simulink model "pts_torque_2"  (Simulink 8.9)
settings: Solver=ode5  StartTime=0.0  StopTime=3.5604  FixedStep=0.005  RelTol=1e-3  AbsTol=1e-6  EnableMultiTasking=on
values from neighbouring files (symbols this model uses):
  Kp = omega.^2    [init_3pts.m]
  kt = [20 7]    [init_3pts.m]
  Kv = 2*chi*omega    [init_3pts.m]
  ListePoints = [130*pi/360 130*pi/360;50*pi/360 90*pi/360; 6*pi/360 60*pi/360]    [init_3pts.m]
undefined symbols (not defined in the file or in its folder): inter_arti_d6, scarabase_ddm, scarabase_dyn
settings Model: SuppressorTable=22 serialization::archive 11 0 6 0 0 0 11 0  Creator=user  LastModifiedBy=steff  ExtModeTrigMode=oneshot  ExtModeArmWhenConnect=off
settings DataIOCC: LimitDataPoints=off  SignalLoggingName=sigsOut
settings OptimizationCC: BooleanDataType=off  ExpressionDepthLimit=2147483647
settings DebuggingCC: SaveWithParameterizedLinksMsg=none  SignalResolutionControl=TryResolveAllWithWarning  MultiTaskDSMMsg=warning  MultiTaskCondExecSysMsg=none
settings HardwareCC: TargetUnknown=on
settings RTWCC: TemplateMakefile=grt_vc.tmf

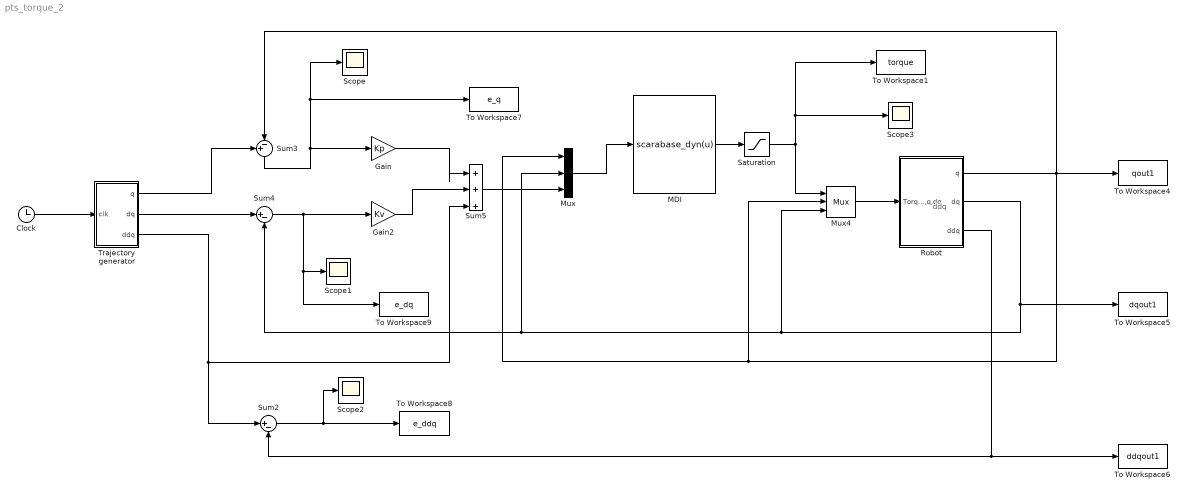
== system pts_torque_2 ==
  note: ddq
  Clock : Clock
  Gain : Gain  Gain=Kp
  Gain2 : Gain  Gain=Kv
  MDI : MATLABFcn  MATLABFcn=scarabase_dyn(u)  OutputDimensions=2  Output1D=off
  Mux : Mux  Inputs=3
  Mux4 : Mux  Inputs=3
  Robot : Subsystem
  Saturation : Saturate  UpperLimit=kt  LowerLimit=-kt
  Scope{,1..3} (4 alike) : Scope
  Sum2 : Sum  Inputs=|+-  SaturateOnIntegerOverflow=on
  Sum3 : Sum  Inputs=+-|  SaturateOnIntegerOverflow=on
  Sum4 : Sum  Inputs=|+-  SaturateOnIntegerOverflow=on
  Sum5 : Sum  Inputs=|+++
  To Workspace1 : ToWorkspace  VariableName=torque  SampleTime=-1
  To Workspace4 : ToWorkspace  VariableName=qout1  SampleTime=-1
  To Workspace5 : ToWorkspace  VariableName=dqout1  SampleTime=-1
  To Workspace6 : ToWorkspace  VariableName=ddqout1  SampleTime=-1
  To Workspace7 : ToWorkspace  VariableName=e_q  SampleTime=-1
  To Workspace8 : ToWorkspace  VariableName=e_ddq  SampleTime=-1
  To Workspace9 : ToWorkspace  VariableName=e_dq  SampleTime=-1
  Trajectory generator : Subsystem
  wires:
  Sum2/1 -> To Workspace8/1, Scope2/1
  Sum3/1 -> Scope/1, To Workspace7/1, Gain/1
  Sum4/1 -> Gain2/1, Scope1/1, To Workspace9/1
  Gain/1 -> Sum5/1
  Gain2/1 -> Sum5/2
  MDI/1 -> Saturation/1
  Mux/1 -> MDI/1
  Saturation/1 -> Mux4/1, To Workspace1/1, Scope3/1
  Sum5/1 -> Mux/3
  Trajectory generator/1(q) -> Sum3/1
  Trajectory generator/3(ddq) -> Sum5/3, Sum2/1
  Trajectory generator/2(dq) -> Sum4/1
  Clock/1 -> Trajectory generator/1(clk)
  Robot/3(ddq) -> Sum2/2, To Workspace6/1
  Robot/2(dq) -> Mux4/3, Mux/2, Sum4/2, To Workspace5/1
  Mux4/1 -> Robot/1(Torque,q,dq)
  Robot/1(q) -> Mux/1, Mux4/2, To Workspace4/1, Sum3/2

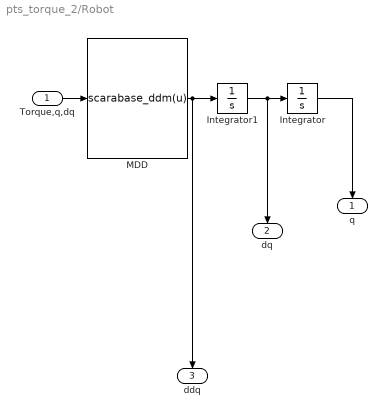
== system pts_torque_2/Robot ==
  Torque,q,dq : Inport
  Integrator : Integrator  InitialCondition=ListePoints(1,:)
  Integrator1 : Integrator  InitialCondition=[0 0]
  MDD : MATLABFcn  MATLABFcn=scarabase_ddm(u)  OutputDimensions=2
  q : Outport
  dq : Outport  Port=2
  ddq : Outport  Port=3
  wires:
  Integrator1/1 -> dq/1, Integrator/1
  Integrator/1 -> q/1
  MDD/1 -> ddq/1, Integrator1/1
  Torque,q,dq/1 -> MDD/1

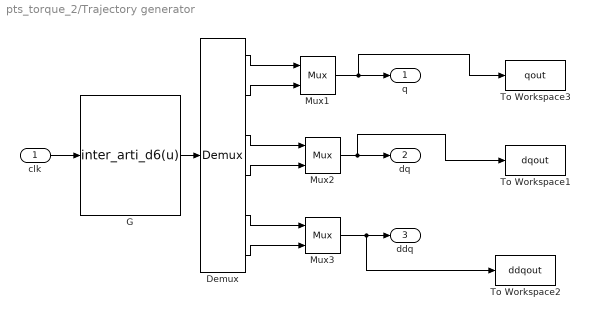
== system pts_torque_2/Trajectory generator ==
  clk : Inport
  Demux : Demux  Outputs=6
  G : MATLABFcn  MATLABFcn=inter_arti_d6(u)  OutputDimensions=6  Output1D=off
  Mux1 : Mux  Inputs=2
  Mux2 : Mux  Inputs=2
  Mux3 : Mux  Inputs=2
  To Workspace1 : ToWorkspace  VariableName=dqout  SampleTime=-1
  To Workspace2 : ToWorkspace  VariableName=ddqout  SampleTime=-1
  To Workspace3 : ToWorkspace  VariableName=qout  SampleTime=-1
  q : Outport
  dq : Outport  Port=2
  ddq : Outport  Port=3
  wires:
  Demux/1 -> Mux1/1
  Demux/6 -> Mux3/2
  Demux/3 -> Mux2/1
  Mux2/1 -> To Workspace1/1, dq/1
  Demux/2 -> Mux1/2
  Demux/4 -> Mux2/2
  Demux/5 -> Mux3/1
  clk/1 -> G/1
  Mux3/1 -> To Workspace2/1, ddq/1
  G/1 -> Demux/1
  Mux1/1 -> To Workspace3/1, q/1
